simulink model "sf_launchabort"  (Simulink 7.6)
settings: Solver=FixedStepDiscrete  SolverMode=SingleTasking  StartTime=0.0  StopTime=136  RelTol=1e-3
values from neighbouring files (symbols this model uses):
  X = get(pi, 'XData')    [sf_edit_icon.m]
undefined symbols (not defined in the file or in its folder): sigbuilder_block
libraries: vrlib x2, simulink x1
CloseFcn:
  | rtwprivate ssgencode ModelCloseRequest launchAbort_phase5
settings Model: Creator=The MathWorks Inc.  CovPath=/launchAbortController  CovMetricSettings=dcmrw
settings OptimizationCC: InitFltsAndDblsToZero=on  EfficientMapNaN2IntZero=off  OptimizeModelRefInitCode=on  LifeSpan=1
settings DebuggingCC: SaveWithParameterizedLinksMsg=none  SignalResolutionControl=TryResolveAllWithWarning  SolverPrmCheckMsg=none  StrictBusMsg=Warning
settings SFSimCC: SimParseCustomCode=off
settings RTWCC: SystemTargetFile=ert.tlc  GenCodeOnly=on  TemplateMakefile=ert_default_tmf  Description=Real-Time Workshop Embedded Coder (no auto configuration)  GenerateReport=on  ProcessScript=ert_make_rtw_hook  IncludeHyperlinkInReport=on  LaunchReport=on
settings CodeAppCC: IgnoreCustomStorageClasses=off  CustomSymbolStrGlobalVar=$N$M  CustomSymbolStrType=$N$M  CustomSymbolStrFcn=$N$M$F  CustomSymbolStrMacro=$N$M
settings ERTTargetCC: TargetFcnLib=ansi_tfl_tmw.mat  MultiwordLength=2048  GenerateSampleERTMain=on  SupportContinuousTime=on  InlinedParameterPlacement=NonHierarchical  ERTCustomFileTemplate=example_file_process.tlc  ConvertIfToSwitch=off

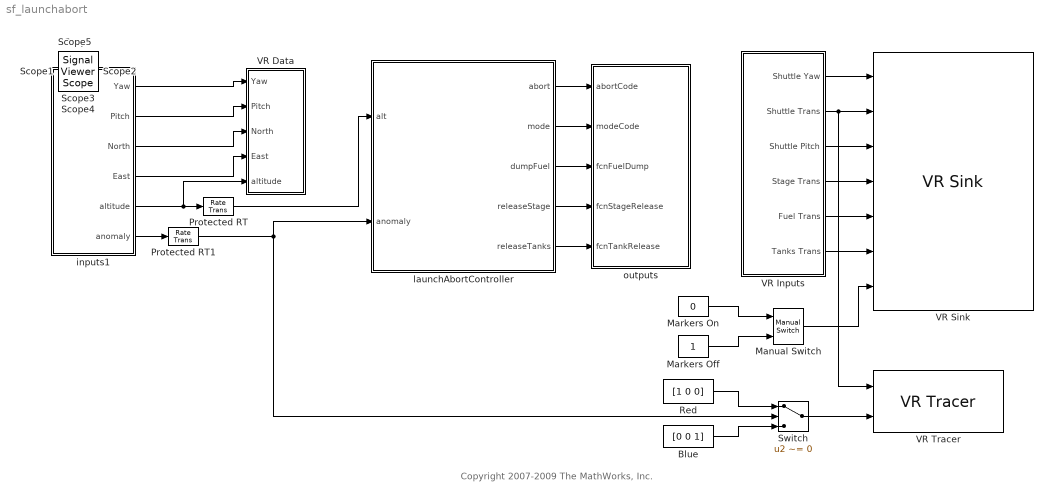
== system sf_launchabort ==
  note: Copyright 2007-2009 The MathWorks, Inc.
  Blue : Constant  Value=[0 0 1]
  Manual Switch : simulink/Signal Routing/Manual Switch  SystemSampleTime=-1  sw=1  action=0  varsize=off
  Markers Off : Constant
  Markers On : Constant  Value=0
  Protected RT : RateTransition  Deterministic=off
  Protected RT1 : RateTransition  Deterministic=off
  Red : Constant  Value=[1 0 0]
  Switch : Switch  Criteria=u2 ~= 0
  VR Data : Subsystem
  VR Inputs : Subsystem
  VR Sink : vrlib/VR Sink  InstantiateOnLoad=on  SampleTime=0.1  ViewEnable=on  RemoteChange=off  RemoteView=on  FieldsWritten=ShuttleYaw.rotation.4.1.double#ShuttleYaw.translation.3.1.double#ShuttlePitch.rotation.4.1.double#StageYaw.translation.3.1.double#dumpedFuel.translation.3.1.double#TanksYaw.translation.3.1.double#Marker_Switch.whichChoice.1.1.double  WorldFileName=abortVR.wrl  WorldDescription=Launch Abort - VR  AutoView=on  VideoDimensions=[]  FigureProperties="{'Position', 'Name', 'Viewpoint', 'CameraBound', 'CameraDirection', 'CameraPosition', 'CameraUpVector', 'ZoomFactor', 'Antialiasing', 'Headlight', 'Lighting', 'NavPanel', 'StatusBar', 'ToolBar', 'Textures', 'Transparency', 'Wireframe', 'NavZones', 'NavMode', 'NavSpeed', 'Record2DCompressMethod', 'Record2DCompressQuality', 'Record2D', 'Record2DFileName', 'Record2DFPS'; [1.1100000000000000e+02   2.6400000000000000e+02   5.8600000000000000e+02   4.0600000000000000e+02], 'Launch Abort - VR', 'Chase Plane', 'on', [0.0000000000000000e+00   0.0000000000000000e+00  -1.0000000000000000e+00], [0.0000000000000000e+00   0.0000000000000000e+00   0.0000000000000000e+00], [0.0000000000000000e+00   1.0000000000000000e+00   0.0000000000000000e+00], [1.0000000000000000e+00], 'on', 'on', 'on', 'halfbar', 'on', 'on', 'on', 'on', 'off', 'off', 'examine', 'veryslow', 'auto', [7.5000000000000000e+01], 'off', '%f_anim_%n.avi', [1.5000000000000000e+01]}"
  VR Tracer : vrlib/VR Tracer  VrmlFile=abortVR.wrl  ParentNode=Markers  MarkerName=Tetrahedron  UseLines=off  UseTriads=off  MarkerScale=[20 20 20]  MarkerColorSelection=Block input  MarkerColor=red  rgbval=[1 0 0]  Ts=1  ForceViewerOpen=off
  inputs1 : Subsystem  Tag=STV Subsys  LoadFcn=sigbuilder_block('load');  StartFcn=sigbuilder_block('start');  StopFcn=sigbuilder_block('stop');  ClipboardFcn=sigbuilder_block('clipboard');  mask(Sigbuilder block){}
      mask help: Sigbuilder GUI
      mask init:
      | if ~strcmp(get_param(bdroot(gcbh),'SimulationStatus'),'stopped') tuvar = sigbuilder_block('maskInit'); end
      settings: CopyFcn=sigbuilder_block('copy');  DeleteFcn=sigbuilder_block('delete');  ModelCloseFcn=sigbuilder_block('modelClose');  PreSaveFcn=sigbuilder_block('preSave');  NameChangeFcn=sigbuilder_block('namechange');  OpenFcn=sigbuilder_block('open',[81 93.75 561 399.75 ]);  CloseFcn=sigbuilder_block('close');
      mask Display: plot(0,0,100,100,[10,10,40,40,10],[80,20,20,80,80],[40,10],[50,50], [40,27,10],[65,72,56],[40,25,25,10],[28,28,43,43]);
  launchAbortController : Stateflow chart  TreatAsAtomicUnit=on
      settings: RTWSystemCode=Reusable function  RTWFcnNameOpts=Use subsystem name  RTWFileNameOpts=Use subsystem name
  outputs : Subsystem
  Scope{,1..5} (6 alike) : SignalViewerScope  IOType=viewer  RefreshTime=0.035000
      Scope2 settings: YMin=-250  YMax=2750  SaveName=ScopeData2
      Scope3 settings: YMin=-250  YMax=2750  SaveName=ScopeData3
      Scope4 settings: YMin=-250  YMax=2750  SaveName=ScopeData4
      Scope5 settings: YMin=0  YMax=60  SaveName=ScopeData5
  wires:
  launchAbortController/1(abort) -> outputs/1(abortCode)
  launchAbortController/2(mode) -> outputs/2(modeCode)
  launchAbortController/3(dumpFuel) -> outputs/3(fcnFuelDump)
  launchAbortController/4(releaseStage) -> outputs/4(fcnStageRelease)
  launchAbortController/5(releaseTanks) -> outputs/5(fcnTankRelease)
  VR Inputs/2(Shuttle Trans) -> VR Sink/2, VR Tracer/1
  inputs1/5(altitude) -> Protected RT/1, VR Data/5(altitude)
  inputs1/4(East) -> VR Data/4(East)
  inputs1/3(North) -> VR Data/3(North)
  inputs1/2(Pitch) -> VR Data/2(Pitch)
  inputs1/1(Yaw) -> VR Data/1(Yaw)
  inputs1/6(anomaly) -> Protected RT1/1
  Protected RT/1 -> launchAbortController/1(alt)
  Protected RT1/1 -> launchAbortController/2(anomaly), Switch/2
  Red/1 -> Switch/1
  Blue/1 -> Switch/3
  VR Inputs/1(Shuttle Yaw) -> VR Sink/1
  VR Inputs/3(Shuttle Pitch) -> VR Sink/3
  VR Inputs/4(Stage Trans) -> VR Sink/4
  VR Inputs/5(Fuel Trans) -> VR Sink/5
  VR Inputs/6(Tanks Trans) -> VR Sink/6
  Markers On/1 -> Manual Switch/1
  Markers Off/1 -> Manual Switch/2
  Manual Switch/1 -> VR Sink/7
  Switch/1 -> VR Tracer/2

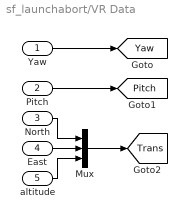
== system sf_launchabort/VR Data ==
  Yaw : Inport
  Pitch : Inport  Port=2
  North : Inport  Port=3
  East : Inport  Port=4
  altitude : Inport  Port=5
  Mux : Mux  Inputs=3
  tag scope: Pitch=global, Trans=global, Yaw=global
  wires:
  East/1 -> Mux/2
  North/1 -> Mux/1
  Pitch/1 -> [Pitch]
  Yaw/1 -> [Yaw]
  altitude/1 -> Mux/3
  Mux/1 -> [Trans]

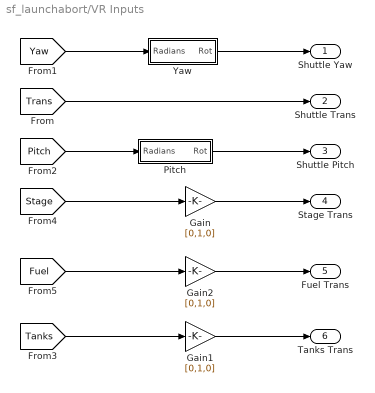
== system sf_launchabort/VR Inputs ==
  Gain : Gain  Gain=[0,1,0]
  Gain1 : Gain  Gain=[0,1,0]
  Gain2 : Gain  Gain=[0,1,0]
  Pitch : Subsystem  mask{axisRot=X}
      mask prompts: axisRot "Axis of Rotation"
      mask StyleString: popup(X|Y|Z)
      mask CallbackString:
      | constantBlock = [gcb, '/rotVector'];
      | switch get_param(gcb, 'axisRot'),
      |     case('X'),
      |         set_param(constantBlock, 'Value', '[1, 0, 0]');
      |     case('Y'),
      |         set_param(constantBlock, 'Value', '[0, 1, 0]');
      |     case('Z'),
      |         set_param(constantBlock, 'Value', '[0, 0, 1]');
      | end
      | clear constantBlock;
  Yaw : Subsystem  mask{axisRot=Z}
      mask prompts: axisRot "Axis of Rotation"
      mask StyleString: popup(X|Y|Z)
      mask CallbackString:
      | constantBlock = [gcb, '/rotVector'];
      | switch get_param(gcb, 'axisRot'),
      |     case('X'),
      |         set_param(constantBlock, 'Value', '[1, 0, 0]');
      |     case('Y'),
      |         set_param(constantBlock, 'Value', '[0, 1, 0]');
      |     case('Z'),
      |         set_param(constantBlock, 'Value', '[0, 0, 1]');
      | end
      | clear constantBlock;
  Shuttle Yaw : Outport
  Shuttle Trans : Outport  Port=2
  Shuttle Pitch : Outport  Port=3
  Stage Trans : Outport  Port=4
  Fuel Trans : Outport  Port=5
  Tanks Trans : Outport  Port=6
  wires:
  [Trans] -> Shuttle Trans/1
  [Tanks] -> Gain1/1
  [Yaw] -> Yaw/1(Radians)
  [Pitch] -> Pitch/1(Radians)
  Pitch/1(Rot) -> Shuttle Pitch/1
  Yaw/1(Rot) -> Shuttle Yaw/1
  Gain/1 -> Stage Trans/1
  Gain1/1 -> Tanks Trans/1
  [Stage] -> Gain/1
  [Fuel] -> Gain2/1
  Gain2/1 -> Fuel Trans/1

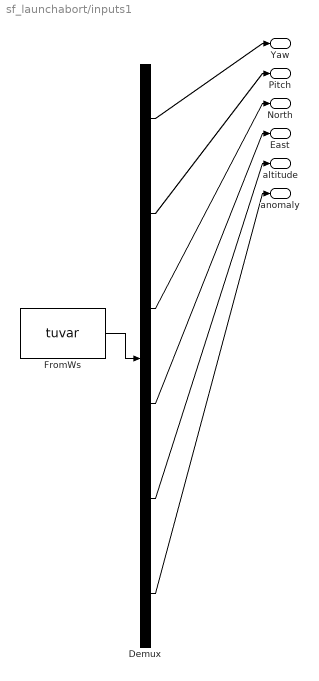
== system sf_launchabort/inputs1 ==
  Demux : Demux  Tag=STV Demux  Outputs=6
  FromWs : FromWorkspace  Tag=STV FromWs  VariableName=tuvar  SampleTime=0  SigBuilderData=DataTag0  VnvData=DataTag1
  Yaw : Outport  Tag=STV Outport
  Pitch : Outport  Tag=STV Outport  Port=2
  North : Outport  Tag=STV Outport  Port=3
  East : Outport  Tag=STV Outport  Port=4
  altitude : Outport  Tag=STV Outport  Port=5
  anomaly : Outport  Tag=STV Outport  Port=6
  wires:
  Demux/6 -> anomaly/1
  Demux/5 -> altitude/1
  Demux/4 -> East/1
  Demux/3 -> North/1
  Demux/2 -> Pitch/1
  Demux/1 -> Yaw/1
  FromWs/1 -> Demux/1

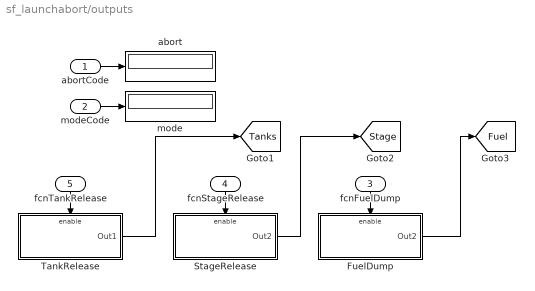
== system sf_launchabort/outputs ==
  abortCode : Inport
  modeCode : Inport  Port=2
  fcnFuelDump : Inport  Port=3
  fcnStageRelease : Inport  Port=4
  fcnTankRelease : Inport  Port=5
  FuelDump : Subsystem  TreatAsAtomicUnit=on
  StageRelease : Subsystem  TreatAsAtomicUnit=on
  TankRelease : Subsystem  TreatAsAtomicUnit=on
  abort : Display
  mode : Display
  tag scope: Fuel=global, Stage=global, Tanks=global
  wires:
  abortCode/1 -> abort/1
  modeCode/1 -> mode/1
  fcnFuelDump/1 -> FuelDump/Enable
  fcnStageRelease/1 -> StageRelease/Enable
  fcnTankRelease/1 -> TankRelease/Enable
  StageRelease/1(Out2) -> [Stage]
  TankRelease/1(Out1) -> [Tanks]
  FuelDump/1(Out2) -> [Fuel]

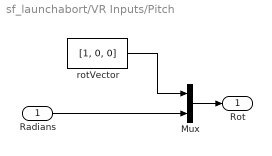
== system sf_launchabort/VR Inputs/Pitch ==
  Radians : Inport
  Mux : Mux  Inputs=2
  rotVector : Constant  Value=[1, 0, 0]
  Rot : Outport
  wires:
  Radians/1 -> Mux/2
  rotVector/1 -> Mux/1
  Mux/1 -> Rot/1

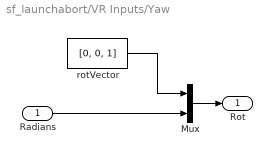
== system sf_launchabort/VR Inputs/Yaw ==
  Radians : Inport
  Mux : Mux  Inputs=2
  rotVector : Constant  Value=[0, 0, 1]
  Rot : Outport
  wires:
  Radians/1 -> Mux/2
  rotVector/1 -> Mux/1
  Mux/1 -> Rot/1

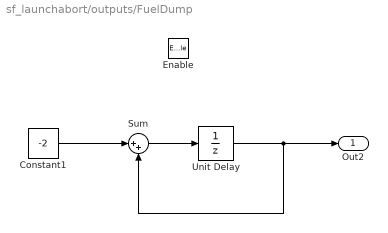
== system sf_launchabort/outputs/FuelDump ==
  Enable : EnablePort
  Constant1 : Constant  Value=-2
  Sum : Sum  Inputs=|++
  Unit Delay : UnitDelay  SampleTime=-1
  Out2 : Outport  InitialOutput=0
  wires:
  Unit Delay/1 -> Sum/2, Out2/1
  Sum/1 -> Unit Delay/1
  Constant1/1 -> Sum/1

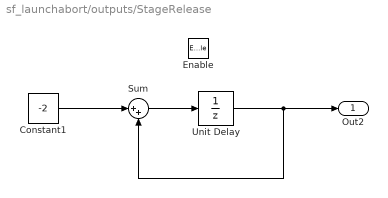
== system sf_launchabort/outputs/StageRelease ==
  Enable : EnablePort
  Constant1 : Constant  Value=-2
  Sum : Sum  Inputs=|++
  Unit Delay : UnitDelay  SampleTime=-1
  Out2 : Outport  InitialOutput=0
  wires:
  Unit Delay/1 -> Sum/2, Out2/1
  Sum/1 -> Unit Delay/1
  Constant1/1 -> Sum/1

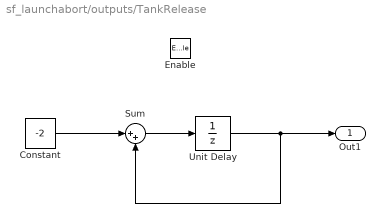
== system sf_launchabort/outputs/TankRelease ==
  Enable : EnablePort
  Constant : Constant  Value=-2
  Sum : Sum  Inputs=|++
  Unit Delay : UnitDelay  SampleTime=-1
  Out1 : Outport  InitialOutput=0
  wires:
  Unit Delay/1 -> Out1/1, Sum/2
  Constant/1 -> Sum/1
  Sum/1 -> Unit Delay/1

== stateflow chart launchAbortController ==
  settings: updateMethod=DISCRETE  sampleTime=1
  state ModeLogic [parallel]
    settings: executionOrder=1
    state ATO
      entry:mode=4;
    state DRL
      entry:mode=2;
    state AOA
      entry:mode=3;
    state RTLS
      entry:mode=1;
    RTLS -> DRL : [alt>10000 && !anomaly]
    DRL -> AOA : [alt>100000 && !anomaly]
    AOA -> ATO : [alt>400000 && !anomaly]
    (default) -> RTLS
  state Abort [parallel]
    settings: executionOrder=2
    state Normal
      en: abort=NO_ABORT;
    state abortLogic
      en: abort = ABORT_STARTED;
      state FuelDump
        dumpFuel;
        ex: abort=FUEL_DUMP_DONE;
      state TankRelease
        releaseTanks;
        ex: abort=TANK_RELEASE_DONE;
      state StageRelease
        releaseStage;
        ex: abort=STAGE_RELEASE_DONE;
      (junction 15) -> FuelDump [order 1] : [in(ModeLogic.RTLS)]
      FuelDump -> TankRelease : after(10, tick)
      (junction 15) -> TankRelease [order 2] : [in(ModeLogic.DRL)]
      (junction 15) -> StageRelease [order 3] : [in(ModeLogic.AOA)]
      (junction 15) -> (junction 16) [order 4]
      TankRelease -> StageRelease : after(10, tick)
      StageRelease -> (junction 16)
    state abortComplete
      en: abort=ABORT_COMPLETE;
    (default) -> Normal
    Normal -> (junction 15) : [anomaly]
    (junction 16) -> abortComplete
  data: alt input double; anomaly input double; abort output double; mode output double; ABORT_COMPLETE constant double =5; ABORT_STARTED constant double =1; FUEL_DUMP_DONE constant double =2; NO_ABORT constant double =0; STAGE_RELEASE_DONE constant double =4; TANK_RELEASE_DONE constant double =3
  events: dumpFuel output EITHER_EDGE_EVENT; releaseStage output EITHER_EDGE_EVENT; releaseTanks output EITHER_EDGE_EVENT
